simulink model "sav2022_opti"  (R2018a)
settings: Solver=VariableStepAuto  StartTime=0  StopTime=30  RelTol=1e-2
settings Model: Creator=tomde  LastModifiedBy=tomde
settings SolverCC: AlgebraicLoopSolver=LineSearch

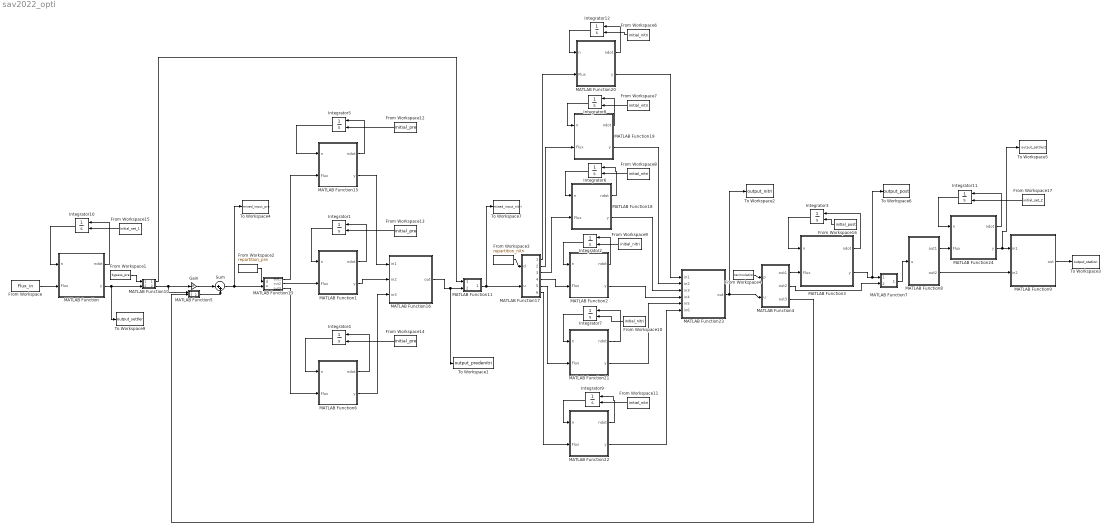
== system sav2022_opti ==
  From Workspace : FromWorkspace  VariableName=Flux_in  OutDataTypeStr=double  SampleTime=0
  From Workspace1 : FromWorkspace  VariableName=bypass_pre  OutDataTypeStr=double  SampleTime=0
  From Workspace{6..11} (6 alike) : FromWorkspace  VariableName=initial_nitri  OutDataTypeStr=double  SampleTime=0
  From Workspace12 : FromWorkspace  VariableName=initial_pre  OutDataTypeStr=double  SampleTime=0
  From Workspace13 : FromWorkspace  VariableName=initial_pre  OutDataTypeStr=double  SampleTime=0
  From Workspace14 : FromWorkspace  VariableName=initial_pre  OutDataTypeStr=double  SampleTime=0
  From Workspace15 : FromWorkspace  VariableName=initial_set_1  OutDataTypeStr=double  SampleTime=0
  From Workspace16 : FromWorkspace  VariableName=initial_post  OutDataTypeStr=double  SampleTime=0
  From Workspace17 : FromWorkspace  VariableName=initial_set_2  OutDataTypeStr=double  SampleTime=0
  From Workspace2 : FromWorkspace  VariableName=repartition_pre  OutDataTypeStr=double  SampleTime=0
  From Workspace3 : FromWorkspace  VariableName=repartition_nitri  OutDataTypeStr=double  SampleTime=0
  From Workspace4 : FromWorkspace  VariableName=recirculation  OutDataTypeStr=double  SampleTime=0
  Gain : Gain  Gain=0
  Integrator{1..12} (12 alike) : Integrator  InitialConditionSource=external  InitialCondition=[122.4 8 25.5 0.018 0.01 43.08 7]
  MATLAB Function : MATLAB Function  TreatAsAtomicUnit=on
  MATLAB Function1 : MATLAB Function  TreatAsAtomicUnit=on
  MATLAB Function10 : MATLAB Function  TreatAsAtomicUnit=on
  MATLAB Function11 : MATLAB Function  TreatAsAtomicUnit=on
  MATLAB Function13 : MATLAB Function  TreatAsAtomicUnit=on
  MATLAB Function15 : MATLAB Function  TreatAsAtomicUnit=on
  MATLAB Function16 : MATLAB Function  TreatAsAtomicUnit=on
  MATLAB Function17 : MATLAB Function  TreatAsAtomicUnit=on
  MATLAB Function18 : MATLAB Function  TreatAsAtomicUnit=on
  MATLAB Function19 : MATLAB Function  TreatAsAtomicUnit=on
  MATLAB Function2 : MATLAB Function  TreatAsAtomicUnit=on
  MATLAB Function20 : MATLAB Function  TreatAsAtomicUnit=on
  MATLAB Function21 : MATLAB Function  TreatAsAtomicUnit=on
  MATLAB Function22 : MATLAB Function  TreatAsAtomicUnit=on
  MATLAB Function23 : MATLAB Function  TreatAsAtomicUnit=on
  MATLAB Function24 : MATLAB Function  TreatAsAtomicUnit=on
  MATLAB Function3 : MATLAB Function  TreatAsAtomicUnit=on
  MATLAB Function4 : MATLAB Function  TreatAsAtomicUnit=on
  MATLAB Function5 : MATLAB Function  TreatAsAtomicUnit=on
  MATLAB Function6 : MATLAB Function  TreatAsAtomicUnit=on
  MATLAB Function7 : MATLAB Function  TreatAsAtomicUnit=on
  MATLAB Function8 : MATLAB Function  TreatAsAtomicUnit=on
  MATLAB Function9 : MATLAB Function  TreatAsAtomicUnit=on
  Sum : Sum  Inputs=|++
  To Workspace1 : ToWorkspace  VariableName=output_predenitri  SaveFormat=Timeseries  SampleTime=-1
  To Workspace2 : ToWorkspace  VariableName=output_nitri  SaveFormat=Timeseries  SampleTime=-1
  To Workspace3 : ToWorkspace  VariableName=output_station  SaveFormat=Timeseries  SampleTime=-1
  To Workspace4 : ToWorkspace  VariableName=mixed_input_pre  SaveFormat=Timeseries  SampleTime=-1
  To Workspace5 : ToWorkspace  VariableName=output_settler2  SaveFormat=Timeseries  SampleTime=-1
  To Workspace6 : ToWorkspace  VariableName=output_post  SaveFormat=Timeseries  SampleTime=-1
  To Workspace7 : ToWorkspace  VariableName=mixed_input_nitri  SaveFormat=Timeseries  SampleTime=-1
  To Workspace9 : ToWorkspace  VariableName=output_settler  SaveFormat=Timeseries  SampleTime=-1
  wires:
  MATLAB Function/1(ndot) -> Integrator10/1
  Integrator10/1 -> MATLAB Function/1(n)
  MATLAB Function10/2(out2) -> MATLAB Function5/1(in1), Gain/1
  MATLAB Function2/1(ndot) -> Integrator2/1
  Integrator2/1 -> MATLAB Function2/1(n)
  Integrator3/1 -> MATLAB Function3/1(n)
  Sum/1 -> To Workspace4/1, MATLAB Function13/2(u)
  MATLAB Function5/1(out) -> Sum/2
  Gain/1 -> Sum/1
  MATLAB Function4/3(out3) -> MATLAB Function5/2(in2)
  MATLAB Function/2(y) -> MATLAB Function10/2(u), To Workspace9/1
  MATLAB Function10/1(out1) -> MATLAB Function11/1(in1)
  From Workspace/1 -> MATLAB Function/2(Flux)
  MATLAB Function13/3(out3) -> MATLAB Function6/2(Flux)
  MATLAB Function13/2(out2) -> MATLAB Function1/2(Flux)
  MATLAB Function15/1(ndot) -> Integrator5/1
  Integrator5/1 -> MATLAB Function15/1(n)
  MATLAB Function13/1(out1) -> MATLAB Function15/2(Flux)
  MATLAB Function15/2(y) -> MATLAB Function16/1(in1)
  MATLAB Function16/1(out) -> To Workspace1/1, MATLAB Function11/2(in2)
  MATLAB Function11/1(out) -> MATLAB Function17/2(u), To Workspace7/1
  MATLAB Function17/4(out4) -> MATLAB Function2/2(Flux)
  Integrator6/1 -> MATLAB Function18/1(n)
  MATLAB Function18/1(ndot) -> Integrator6/1
  Integrator8/1 -> MATLAB Function19/1(n)
  MATLAB Function19/1(ndot) -> Integrator8/1
  MATLAB Function20/1(ndot) -> Integrator12/1
  Integrator12/1 -> MATLAB Function20/1(n)
  Integrator7/1 -> MATLAB Function21/1(n)
  MATLAB Function21/1(ndot) -> Integrator7/1
  Integrator9/1 -> MATLAB Function22/1(n)
  MATLAB Function22/1(ndot) -> Integrator9/1
  MATLAB Function17/3(out3) -> MATLAB Function18/2(Flux)
  MATLAB Function17/2(out2) -> MATLAB Function19/2(Flux)
  MATLAB Function17/1(out1) -> MATLAB Function20/2(Flux)
  MATLAB Function17/5(out5) -> MATLAB Function21/2(Flux)
  MATLAB Function17/6(out6) -> MATLAB Function22/2(Flux)
  MATLAB Function2/2(y) -> MATLAB Function23/4(in4)
  MATLAB Function21/2(y) -> MATLAB Function23/5(in5)
  MATLAB Function22/2(y) -> MATLAB Function23/6(in6)
  MATLAB Function18/2(y) -> MATLAB Function23/3(in3)
  MATLAB Function19/2(y) -> MATLAB Function23/2(in2)
  MATLAB Function20/2(y) -> MATLAB Function23/1(in1)
  MATLAB Function23/1(out) -> To Workspace2/1, MATLAB Function4/2(u)
  MATLAB Function24/1(ndot) -> Integrator11/1
  Integrator11/1 -> MATLAB Function24/1(n)
  MATLAB Function24/2(y) -> To Workspace5/1, MATLAB Function9/1(in1)
  MATLAB Function4/1(out1) -> MATLAB Function3/2(Flux)
  MATLAB Function8/1(out1) -> MATLAB Function24/2(Flux)
  MATLAB Function8/2(out2) -> MATLAB Function9/2(in2)
  Integrator1/1 -> MATLAB Function1/1(n)
  MATLAB Function1/1(ndot) -> Integrator1/1
  Integrator4/1 -> MATLAB Function6/1(n)
  MATLAB Function6/1(ndot) -> Integrator4/1
  MATLAB Function1/2(y) -> MATLAB Function16/2(in2)
  MATLAB Function6/2(y) -> MATLAB Function16/3(in3)
  From Workspace1/1 -> MATLAB Function10/1(p)
  From Workspace2/1 -> MATLAB Function13/1(d)
  From Workspace3/1 -> MATLAB Function17/1(d)
  From Workspace4/1 -> MATLAB Function4/1(p)
  From Workspace6/1 -> Integrator12/2
  From Workspace7/1 -> Integrator8/2
  From Workspace8/1 -> Integrator6/2
  From Workspace9/1 -> Integrator2/2
  From Workspace10/1 -> Integrator7/2
  From Workspace11/1 -> Integrator9/2
  From Workspace12/1 -> Integrator5/2
  From Workspace13/1 -> Integrator1/2
  From Workspace14/1 -> Integrator4/2
  From Workspace15/1 -> Integrator10/2
  From Workspace16/1 -> Integrator3/2
  MATLAB Function3/1(ndot) -> Integrator3/1
  From Workspace17/1 -> Integrator11/2
  MATLAB Function9/1(out) -> To Workspace3/1
  MATLAB Function4/2(out2) -> MATLAB Function7/2(in2)
  MATLAB Function3/2(y) -> To Workspace6/1, MATLAB Function7/1(in1)
  MATLAB Function7/1(out) -> MATLAB Function8/1(u)

== matlab function sav2022_opti/MATLAB Function1 ==
  data: ndot output; n input; Flux input; y output
function [ndot,y] = pre_denitrification(n,Flux)
Y=[0.675 0.297 2.3];
mu=[3.95 1.99];

K_NO3_1=0.4;
K_NO2_1=1.05;
K_COD_1=71.5;
K_COD_2=11.6;
X1=465.6;
V2=35090/3;


C_in=Flux(1:8);
Q =Flux(8);

dndt=zeros(7,1);
dndt(1)=Q/V2*(C_in(1)-n(1));
dndt(2)=Q/V2*(C_in(2)-n(2));
dndt(3)=-1/Y(1)*mu(1)*n(6)/(K_NO3_1+n(6))*n(3)/(K_COD_1+n(3))*X1-1/Y(2)*mu(2)*n(5)/(K_NO2_1+n(5))*n(3)/(K_COD_2+n(3))*X1+Q/V2*(C_in(3)-n(3));
dndt(4)=Q/V2*(C_in(4)-n(4));
dndt(5)=1/Y(3)*mu(1)*n(6)/(K_NO3_1+n(6))*n(3)/(K_COD_1+n(3))*X1-mu(2)*n(5)/(K_NO2_1+n(5))*n(3)/(K_COD_2+n(3))*X1+Q/V2*(C_in(5)-n(5));
dndt(6)=-mu(1)*n(6)/(K_NO3_1+n(6))*n(3)/(K_COD_1+n(3))*X1+Q/V2*(C_in(6)-n(6));
dndt(7)=Q/V2*(C_in(7)-n(7));
if n(3)<10^(-6)
    n(3)=0;
end
if n(6)<10^(-6)
    n(6)=0;
end
if n(5)<10^(-6)
    n(5)=0;
end

if n(4)<10^(-6)
    n(4)=0;
end

ndot = dndt;
y=[n;Q];
end

== matlab function sav2022_opti/MATLAB Function ==
  data: ndot output; n input; Flux input; y output
function [ndot,y] = settler(n,Flux)

 k=[256.76 2.6643 2.2693];

 K_FeCl3=0.000001;
 K_PO4=0.0346;

V1=32445;
C_in=Flux(1:7);
Q =Flux(8);
u_r=[32.6 0]; %FeCl3 [g/m^3]
dndt=zeros(7,1);
 % interp1(T, Q_in, t);
dndt(1)=-k(1)*n(1)*u_r(1)/(K_FeCl3+u_r(1)) + Q/V1*(C_in(1)-n(1)); %TSS removal
dndt(2)=-k(2)*n(2)*u_r(1)/(K_PO4+n(2)) + Q/V1*(C_in(2)-n(2));
dndt(3)=-k(3)*n(3)*u_r(1)+Q/V1*(C_in(3)-n(3));
dndt(4)=Q/V1*(C_in(4)-n(4));
dndt(5)=Q/V1*(C_in(5)-n(5));
dndt(6)=Q/V1*(C_in(6)-n(6));
dndt(7)=Q/V1*(C_in(7)-n(7));

if n(1)<10^(-6)
    n(1)=0;
end
if n(2)<10^(-6)
    n(2)=0;
end
if n(3)<10^(-6)
    n(3)=0;
end
ndot = dndt;
y=[n;Q];
end

== matlab function sav2022_opti/MATLAB Function2 ==
  data: ndot output; n input; Flux input; y output
function [ndot,y] = Nitrification(n,Flux)
Y=[1.67 0.16];
mu=[0.072 50.8 1.67 0.88 576.97 0.31];

K_NO2_2=0.01;
K_NH4=0.01;
K_O2_1=1.501E-4;
K_O2_2=4.42E-13;


X2=640;
X3=634;



V3=50820/6;

C_in=Flux(1:7);
Q =Flux(8);

dndt=zeros(7,1);
dndt(1)=Q/V3*(C_in(1)-n(1));
dndt(2)=Q/V3*(C_in(2)-n(2));
dndt(3)=Q/V3*(C_in(3)-n(3));
dndt(4)=-mu(3)*n(4)/(K_NH4+n(4))*X2+Q/V3*(C_in(4)-n(4));
dndt(5)=1/Y(1)*mu(3)*n(4)/(K_NH4+n(4))*X2-mu(4)*n(5)/(K_NO2_2+n(5))*X3+Q/V3*(C_in(5)-n(5));
dndt(6)=1/Y(2)*mu(4)*n(5)/(K_NO2_2+n(5))*n(7)/(K_O2_2+n(7))*X3+Q/V3*(C_in(6)-n(6));
dndt(7)=0;%-1/Y(6)*mu(3)*n(4)/(K_NH4+n(4))*n(7)/(K_O2_2+n(7))*X2-1/Y(7)*mu(4)*n(6)/(K_NO2_2+n(6))*n(7)/(K_O2_2+n(7))*X3+Q/V3*(C_in(7)-n(7));
if n(6)<10^(-6)
    n(6)=0;
end
if n(4)<10^(-6)
    n(4)=0;
end
if n(5)<10^(-6)
    n(5)=0;
end
ndot = dndt;
y=[n;Q];
end

== matlab function sav2022_opti/MATLAB Function3 ==
  data: ndot output; n input; Flux input; y output
function [ndot,y] = post_denitrification(n,Flux)
Y=[0.077 0.14 40.57 6.87 0.14 3.19*10^5 1.67*10^5 0.25 0.96 27.57];
mu=[0.072 50.8 1.67 0.88 11.6 9.4];


K_NO3_2=0.1;
K_NO2_3=4.42E-8;
K_COD_3=70.29;
K_COD_4=0.001;



X4=582;

V4=16182;

C_in=Flux(1:7);
Q =Flux(8);


dndt=zeros(7,1);
dndt(1)=Q/V4*(C_in(1)-n(1));
dndt(2)=Q/V4*(C_in(2)-n(2));
dndt(3)=-1/Y(8)*mu(5)*n(6)/(K_NO3_2+n(6))*n(3)/(K_COD_3+n(3))*X4-1/Y(9)*mu(6)*n(5)/(K_NO2_3+n(5))*n(3)/(K_COD_4+n(3))+Q/V4*(C_in(3)-n(3));
dndt(4)=Q/V4*(C_in(4)-n(4));
dndt(5)=1/Y(10)*mu(5)*n(6)/(K_NO3_2+n(6))*n(3)/(K_COD_3+n(3))*X4-mu(6)*n(5)/(K_NO2_3+n(5))*n(3)/(K_COD_4+n(3))+Q/V4*(C_in(5)-n(5));
dndt(6)=-mu(5)*n(6)/(K_NO3_2+n(6))*n(3)/(K_COD_3+n(3))*X4+Q/V4*(C_in(6)-n(6));
dndt(7)=Q/V4*(C_in(7)-n(7));
if n(6)<10^(-6)
    n(6)=0;
end
if n(3)<10^(-6)
    n(3)=0;
end
if n(5)<10^(-6)
    n(5)=0;
end
ndot = dndt;
y=[n;Q];
end

== matlab function sav2022_opti/MATLAB Function4 ==
  data: p input; u input; out1 output; out2 output; out3 output

function [out1,out2,out3] = fcn(p,u)
if u(8)-p>11.2*3600*24
out1=[u(1:7);11.2*3600*24];
out2=[u(1:7);u(8)-p-11.2*3600*24];
out3=[u(1:7);p];
else
out1=[u(1:7);u(8)-p];
out2=[u(1:7);0];
out3=[u(1:7);p];   
end

end

== matlab function sav2022_opti/MATLAB Function5 ==
  data: in1 input; out output; in2 input

function out  = SUM(in1,in2)



C=(in1(1:7).*in1(8)+in2(1:7).*in2(8))./(in1(8)+in2(8));
Q=in1(8)+in2(8);
out=[C;Q];

end

== matlab function sav2022_opti/MATLAB Function6 ==
  data: ndot output; n input; Flux input; y output
function [ndot,y] = pre_denitrification(n,Flux)
Y=[0.675 0.297 2.3];
mu=[3.95 1.99];

K_NO3_1=0.4;
K_NO2_1=1.05;
K_COD_1=71.5;
K_COD_2=11.6;
X1=465.6;
V2=35090/3;


C_in=Flux(1:8);
Q =Flux(8);

dndt=zeros(7,1);
dndt(1)=Q/V2*(C_in(1)-n(1));
dndt(2)=Q/V2*(C_in(2)-n(2));
dndt(3)=-1/Y(1)*mu(1)*n(6)/(K_NO3_1+n(6))*n(3)/(K_COD_1+n(3))*X1-1/Y(2)*mu(2)*n(5)/(K_NO2_1+n(5))*n(3)/(K_COD_2+n(3))*X1+Q/V2*(C_in(3)-n(3));
dndt(4)=Q/V2*(C_in(4)-n(4));
dndt(5)=1/Y(3)*mu(1)*n(6)/(K_NO3_1+n(6))*n(3)/(K_COD_1+n(3))*X1-mu(2)*n(5)/(K_NO2_1+n(5))*n(3)/(K_COD_2+n(3))*X1+Q/V2*(C_in(5)-n(5));
dndt(6)=-mu(1)*n(6)/(K_NO3_1+n(6))*n(3)/(K_COD_1+n(3))*X1+Q/V2*(C_in(6)-n(6));
dndt(7)=Q/V2*(C_in(7)-n(7));
if n(3)<10^(-6)
    n(3)=0;
end
if n(6)<10^(-6)
    n(6)=0;
end
if n(5)<10^(-6)
    n(5)=0;
end

if n(4)<10^(-6)
    n(4)=0;
end

ndot = dndt;
y=[n;Q];
end

== matlab function sav2022_opti/MATLAB Function7 ==
  data: in1 input; out output; in2 input

function out  = SUM(in1,in2)



C=(in1(1:7).*in1(8)+in2(1:7).*in2(8))./(in1(8)+in2(8));
Q=in1(8)+in2(8);
out=[C;Q];

end

== matlab function sav2022_opti/MATLAB Function8 ==
  data: u input; out1 output; out2 output

function [out1,out2] = fcn(u)
if u(8)>25*3600*24
out1=[u(1:7);25*3600*24];
out2=[u(1:7);u(8)-25*3600*24];
else
  out1=[u(1:7);u(8)];
out2=[u(1:7);0];  
end


end

== matlab function sav2022_opti/MATLAB Function9 ==
  data: in1 input; out output; in2 input

function out  = SUM(in1,in2)



C=(in1(1:7).*in1(8)+in2(1:7).*in2(8))./(in1(8)+in2(8));
Q=in1(8)+in2(8);
out=[C;Q];

end

== matlab function sav2022_opti/MATLAB Function10 ==
  data: p input; u input; out1 output; out2 output

function [out1,out2] = fcn(p,u)
out2=[u(1:7);u(8)-p];
out1=[u(1:7);p];

end

== matlab function sav2022_opti/MATLAB Function11 ==
  data: in1 input; out output; in2 input

function out  = SUM(in1,in2)



C=(in1(1:7).*in1(8)+in2(1:7).*in2(8))./(in1(8)+in2(8));
Q=in1(8)+in2(8);
out=[C;Q];

end

== matlab function sav2022_opti/MATLAB Function13 ==
  data: d input; u input; out1 output; out2 output; out3 output

function [out1,out2,out3] = fcn(d,u)

out1=[u(1:7);d(1)];
out2=[u(1:7);d(2)];
out3=[u(1:7);d(3)];
end

== matlab function sav2022_opti/MATLAB Function15 ==
  data: ndot output; n input; Flux input; y output
function [ndot,y] = pre_denitrification(n,Flux)
Y=[0.675 0.297 2.3];
mu=[3.95 1.99];

K_NO3_1=0.4;
K_NO2_1=1.05;
K_COD_1=71.5;
K_COD_2=11.6;
X1=465.6;
V2=35090/3;


C_in=Flux(1:8);
Q =Flux(8);

dndt=zeros(7,1);
dndt(1)=Q/V2*(C_in(1)-n(1));
dndt(2)=Q/V2*(C_in(2)-n(2));
dndt(3)=-1/Y(1)*mu(1)*n(6)/(K_NO3_1+n(6))*n(3)/(K_COD_1+n(3))*X1-1/Y(2)*mu(2)*n(5)/(K_NO2_1+n(5))*n(3)/(K_COD_2+n(3))*X1+Q/V2*(C_in(3)-n(3));
dndt(4)=Q/V2*(C_in(4)-n(4));
dndt(5)=1/Y(3)*mu(1)*n(6)/(K_NO3_1+n(6))*n(3)/(K_COD_1+n(3))*X1-mu(2)*n(5)/(K_NO2_1+n(5))*n(3)/(K_COD_2+n(3))*X1+Q/V2*(C_in(5)-n(5));
dndt(6)=-mu(1)*n(6)/(K_NO3_1+n(6))*n(3)/(K_COD_1+n(3))*X1+Q/V2*(C_in(6)-n(6));
dndt(7)=Q/V2*(C_in(7)-n(7));
if n(3)<10^(-6)
    n(3)=0;
end
if n(6)<10^(-6)
    n(6)=0;
end
if n(5)<10^(-6)
    n(5)=0;
end

if n(4)<10^(-6)
    n(4)=0;
end

ndot = dndt;
y=[n;Q];
end

== matlab function sav2022_opti/MATLAB Function16 ==
  data: in1 input; out output; in2 input; in3 input

function out  = SUM(in1,in2,in3)

if in1(8)==0 && in2(8)==0 && in3(8)==0 
    out=[in1(1:7);0];
else

C=(in1(1:7).*in1(8)+in2(1:7).*in2(8)+in3(1:7).*in3(8))./(in1(8)+in2(8)+in3(8));
Q=in1(8)+in2(8)+in3(8);
out=[C;Q];
end
end

== matlab function sav2022_opti/MATLAB Function17 ==
  data: d input; u input; out1 output; out2 output; out3 output; out4 output; out5 output; out6 output

function [out1,out2,out3,out4,out5,out6] = fcn(d,u)

out1=[u(1:7);d(1)];
out2=[u(1:7);d(2)];
out3=[u(1:7);d(3)];
out4=[u(1:7);d(4)];
out5=[u(1:7);d(5)];
out6=[u(1:7);d(6)];
end

== matlab function sav2022_opti/MATLAB Function18 ==
  data: ndot output; n input; Flux input; y output
function [ndot,y] = Nitrification(n,Flux)
Y=[1.67 0.16];
mu=[0.072 50.8 1.67 0.88 576.97 0.31];

K_NO2_2=0.01;
K_NH4=0.01;
K_O2_1=1.501E-4;
K_O2_2=4.42E-13;


X2=640;
X3=634;



V3=50820/6;

C_in=Flux(1:7);
Q =Flux(8);

dndt=zeros(7,1);
dndt(1)=Q/V3*(C_in(1)-n(1));
dndt(2)=Q/V3*(C_in(2)-n(2));
dndt(3)=Q/V3*(C_in(3)-n(3));
dndt(4)=-mu(3)*n(4)/(K_NH4+n(4))*X2+Q/V3*(C_in(4)-n(4));
dndt(5)=1/Y(1)*mu(3)*n(4)/(K_NH4+n(4))*X2-mu(4)*n(5)/(K_NO2_2+n(5))*X3+Q/V3*(C_in(5)-n(5));
dndt(6)=1/Y(2)*mu(4)*n(5)/(K_NO2_2+n(5))*n(7)/(K_O2_2+n(7))*X3+Q/V3*(C_in(6)-n(6));
dndt(7)=0;%-1/Y(6)*mu(3)*n(4)/(K_NH4+n(4))*n(7)/(K_O2_2+n(7))*X2-1/Y(7)*mu(4)*n(6)/(K_NO2_2+n(6))*n(7)/(K_O2_2+n(7))*X3+Q/V3*(C_in(7)-n(7));
if n(6)<10^(-6)
    n(6)=0;
end
if n(4)<10^(-6)
    n(4)=0;
end
if n(5)<10^(-6)
    n(5)=0;
end
ndot = dndt;
y=[n;Q];
end

== matlab function sav2022_opti/MATLAB Function19 ==
  data: ndot output; n input; Flux input; y output
function [ndot,y] = Nitrification(n,Flux)
Y=[1.67 0.16];

mu=[0.072 50.8 1.67 0.88 576.97 0.31];

K_NO2_2=0.01;
K_NH4=0.01;
K_O2_1=1.501E-4;
K_O2_2=4.42E-13;


X2=640;
X3=634;



V3=50820/6;

C_in=Flux(1:7);
Q =Flux(8);

dndt=zeros(7,1);
dndt(1)=Q/V3*(C_in(1)-n(1));
dndt(2)=Q/V3*(C_in(2)-n(2));
dndt(3)=Q/V3*(C_in(3)-n(3));
dndt(4)=-mu(3)*n(4)/(K_NH4+n(4))*X2+Q/V3*(C_in(4)-n(4));
dndt(5)=1/Y(1)*mu(3)*n(4)/(K_NH4+n(4))*X2-mu(4)*n(5)/(K_NO2_2+n(5))*X3+Q/V3*(C_in(5)-n(5));
dndt(6)=1/Y(2)*mu(4)*n(5)/(K_NO2_2+n(5))*n(7)/(K_O2_2+n(7))*X3+Q/V3*(C_in(6)-n(6));
dndt(7)=0;%-1/Y(6)*mu(3)*n(4)/(K_NH4+n(4))*n(7)/(K_O2_2+n(7))*X2-1/Y(7)*mu(4)*n(6)/(K_NO2_2+n(6))*n(7)/(K_O2_2+n(7))*X3+Q/V3*(C_in(7)-n(7));
if n(6)<10^(-6)
    n(6)=0;
end
if n(4)<10^(-6)
    n(4)=0;
end
if n(5)<10^(-6)
    n(5)=0;
end
ndot = dndt;
y=[n;Q];
end

== matlab function sav2022_opti/MATLAB Function20 ==
  data: ndot output; n input; Flux input; y output
function [ndot,y] = Nitrification(n,Flux)
Y4=1.67;

Y5=0.16;
mu3=1.67;
mu4=0.88;

K_NO2_2=0.01;
K_NH4=0.01;


X2=640;
X3=634;



V3=50820/6;

C_in=Flux(1:7);
Q =Flux(8);

dndt=zeros(7,1);
dndt(1)=Q/V3*(C_in(1)-n(1));
dndt(2)=Q/V3*(C_in(2)-n(2));
dndt(3)=Q/V3*(C_in(3)-n(3));
dndt(4)=-mu3*n(4)/(K_NH4+n(4))*X2+Q/V3*(C_in(4)-n(4));
dndt(5)=1/Y4*mu3*n(4)/(K_NH4+n(4))*X2-mu4*n(5)/(K_NO2_2+n(5))*X3+Q/V3*(C_in(5)-n(5));
dndt(6)=1/Y5*mu4*n(5)/(K_NO2_2+n(5))*X3+Q/V3*(C_in(6)-n(6));
dndt(7)=0;%-1/Y(6)*mu(3)*n(4)/(K_NH4+n(4))*n(7)/(K_O2_2+n(7))*X2-1/Y(7)*mu(4)*n(6)/(K_NO2_2+n(6))*n(7)/(K_O2_2+n(7))*X3+Q/V3*(C_in(7)-n(7));
if n(6)<10^(-6)
    n(6)=0;
end
if n(4)<10^(-6)
    n(4)=0;
end
if n(5)<10^(-6)
    n(5)=0;
end
ndot = dndt;
y=[n;Q];
end

== matlab function sav2022_opti/MATLAB Function21 ==
  data: ndot output; n input; Flux input; y output
function [ndot,y] = Nitrification(n,Flux)
Y=[1.67 0.16];
mu=[0.072 50.8 1.67 0.88 576.97 0.31];

K_NO2_2=0.01;
K_NH4=0.01;
K_O2_1=1.501E-4;
K_O2_2=4.42E-13;


X2=640;
X3=634;



V3=50820/6;

C_in=Flux(1:7);
Q =Flux(8);

dndt=zeros(7,1);
dndt(1)=Q/V3*(C_in(1)-n(1));
dndt(2)=Q/V3*(C_in(2)-n(2));
dndt(3)=Q/V3*(C_in(3)-n(3));
dndt(4)=-mu(3)*n(4)/(K_NH4+n(4))*X2+Q/V3*(C_in(4)-n(4));
dndt(5)=1/Y(1)*mu(3)*n(4)/(K_NH4+n(4))*X2-mu(4)*n(5)/(K_NO2_2+n(5))*X3+Q/V3*(C_in(5)-n(5));
dndt(6)=1/Y(2)*mu(4)*n(5)/(K_NO2_2+n(5))*n(7)/(K_O2_2+n(7))*X3+Q/V3*(C_in(6)-n(6));
dndt(7)=0;%-1/Y(6)*mu(3)*n(4)/(K_NH4+n(4))*n(7)/(K_O2_2+n(7))*X2-1/Y(7)*mu(4)*n(6)/(K_NO2_2+n(6))*n(7)/(K_O2_2+n(7))*X3+Q/V3*(C_in(7)-n(7));
if n(6)<10^(-6)
    n(6)=0;
end
if n(4)<10^(-6)
    n(4)=0;
end
if n(5)<10^(-6)
    n(5)=0;
end
ndot = dndt;
y=[n;Q];
end

== matlab function sav2022_opti/MATLAB Function22 ==
  data: ndot output; n input; Flux input; y output
function [ndot,y] = Nitrification(n,Flux)
Y=[1.67 0.16];
mu=[0.072 50.8 1.67 0.88 576.97 0.31];

K_NO2_2=0.01;
K_NH4=0.01;
K_O2_1=1.501E-4;
K_O2_2=4.42E-13;


X2=640;
X3=634;



V3=50820/6;

C_in=Flux(1:7);
Q =Flux(8);

dndt=zeros(7,1);
dndt(1)=Q/V3*(C_in(1)-n(1));
dndt(2)=Q/V3*(C_in(2)-n(2));
dndt(3)=Q/V3*(C_in(3)-n(3));
dndt(4)=-mu(3)*n(4)/(K_NH4+n(4))*X2+Q/V3*(C_in(4)-n(4));
dndt(5)=1/Y(1)*mu(3)*n(4)/(K_NH4+n(4))*X2-mu(4)*n(5)/(K_NO2_2+n(5))*X3+Q/V3*(C_in(5)-n(5));
dndt(6)=1/Y(2)*mu(4)*n(5)/(K_NO2_2+n(5))*n(7)/(K_O2_2+n(7))*X3+Q/V3*(C_in(6)-n(6));
dndt(7)=0;%-1/Y(6)*mu(3)*n(4)/(K_NH4+n(4))*n(7)/(K_O2_2+n(7))*X2-1/Y(7)*mu(4)*n(6)/(K_NO2_2+n(6))*n(7)/(K_O2_2+n(7))*X3+Q/V3*(C_in(7)-n(7));

if n(6)<10^(-6)
    n(6)=0;
end
if n(4)<10^(-6)
    n(4)=0;
end
if n(5)<10^(-6)
    n(5)=0;
end
ndot = dndt;
y=[n;Q];
end

== matlab function sav2022_opti/MATLAB Function23 ==
  data: in1 input; out output; in2 input; in3 input; in4 input; in5 input; in6 input

function out  = SUM(in1,in2,in3,in4,in5,in6)

if in1(8)==0 && in2(8)==0 && in3(8)==0 && in4(8)==0 && in5(8)==0 && in6(8)==0
    out=[in1(1:7);0];
else

C=(in1(1:7).*in1(8)+in2(1:7).*in2(8)+in3(1:7).*in3(8)+in4(1:7).*in4(8)+in5(1:7).*in5(8)+in6(1:7).*in6(8))./(in1(8)+in2(8)+in3(8)+in4(8)+in5(8)+in6(8));
Q=in1(8)+in2(8)+in3(8)+in4(8)+in5(8)+in6(8);
out=[C;Q];
end
end

== matlab function sav2022_opti/MATLAB Function24 ==
  data: ndot output; n input; Flux input; y output
function [ndot,y] = settler(n,Flux)

  k=[256.76 2.6643 2.2693];

 K_FeCl3=0.000001;
 K_PO4=0.0346;

V1=34704;
C_in=Flux(1:7);
Q =Flux(8);
u_r=[32.6 0]; %FeCl3 [g/m^3]
dndt=zeros(7,1);
 % interp1(T, Q_in, t);
dndt(1)=-k(1)*n(1)*u_r(1)/(K_FeCl3+u_r(1)) + Q/V1*(C_in(1)-n(1)); %TSS removal
dndt(2)=-k(2)*n(2)*u_r(1)/(K_PO4+n(2)) + Q/V1*(C_in(2)-n(2));
dndt(3)=-k(3)*n(3)*u_r(1)+Q/V1*(C_in(3)-n(3));
dndt(4)=Q/V1*(C_in(4)-n(4));
dndt(5)=Q/V1*(C_in(5)-n(5));
dndt(6)=Q/V1*(C_in(6)-n(6));
dndt(7)=Q/V1*(C_in(7)-n(7));

if n(1)<10^(-6)
    n(1)=0;
end
if n(2)<10^(-6)
    n(2)=0;
end
if n(3)<10^(-6)
    n(3)=0;
end
ndot = dndt;
y=[n;Q];
end
